simulink model "Hexa_CAD_ANSFT_Sim_V2"  (R2024b)
settings: Solver=ode4  StartTime=0.0  StopTime=30  FixedStep=0.01  RelTol=1e-3
model workspace (MAT data in the model file):
  hover_2m = [0 0 2 0 0 0 0 0 2 0 0 0 ... (36 elements, 6x6)]
  square = [0 0 2.5 0 0 0 0 0 2.5 0 0 0 ... (36 elements, 6x6)]
  tf : Simulink.Parameter (value not decoded)
  tray0 = [0 0 0 0 0 0 0.2 0.15 2 0 0 0 ... (36 elements, 6x6)]
  tray1 = [0 0 0 0 0 0 0 0 2 0 0 0 ... (36 elements, 6x6)]
  tray2 = [0 0 0 0 0 0 2 0 5 0 0 0 ... (36 elements, 6x6)]
  tray3 = [0 0 0 0 0 0 2 0 5 0 0 0 ... (36 elements, 6x6)]
  tray4 = [0 0 0 0 0 0 2 0 5 0.15 0 0 ... (36 elements, 6x6)]
  tray5 = [0 0 0 0 0 0 0 0 5 0.15 0 0 ... (36 elements, 6x6)]
  tray_yaw = [0 0 0 0 0 0 0 0 5 0 0 0 ... (36 elements, 6x6)]
undefined symbols (not defined in the file or in its folder): F, Light, MIL, smiData, X, Y, Z
libraries: sm_lib x167, nesl_utility x29, dspobslib x9, simulink x5, sharedtransform x2, robotcorelib x1, aerolibwind2 x1
(part 6 of 6)

== matlab function Hexa_CAD_ANSFT_Sim_V2/Controller/Rib function ==
  data: pose input; Rbi output
function Rbi  = fcn(pose)

%% Rib matrix calculation

roll = pose(4);
pitch = pose(5);
yaw = pose(6);

R1 = [cos(yaw)*cos(pitch), -cos(roll)*sin(yaw) + cos(yaw)*sin(roll)*sin(pitch), sin(roll)*sin(yaw) + cos(roll)*cos(yaw)*sin(pitch);
       cos(pitch)*sin(yaw), cos(roll)*cos(yaw) + sin(yaw)*sin(pitch)*sin(roll), -cos(yaw)*sin(roll) + sin(yaw)*sin(pitch)*cos(roll);
       -sin(pitch), cos(pitch)*sin(roll), cos(pitch)*cos(roll)];

R2 = [1, sin(roll)*tan(pitch), cos(roll)*tan(pitch);
      0, cos(roll), -sin(roll);
      0, sin(roll)/cos(pitch), cos(roll)/cos(pitch)];

Rzeros = zeros(3);

Rib = [R1, Rzeros;
       Rzeros, R2];
Rbi = inv(Rib);

== matlab function Hexa_CAD_ANSFT_Sim_V2/6DoF_Dynamics/calculatePWM ==
  data: omega2 input; pwm output
function pwm = fcn(omega2)

pwm = -1.935e-09 .* omega2 .* omega2 + 0.001723 .* omega2 + 1114.0412;
